simulink model "AKZkz"  (Simulink 4.00)
settings: Solver=ode23tb  StartTime=0.0  StopTime=1
InitFcn:
  | powericon('psbinitsys',bdroot);
libraries: powerlib2 x3, powerlib_extras x3
settings Model: LastModifiedBy=ieao  BlockReductionOpt=off

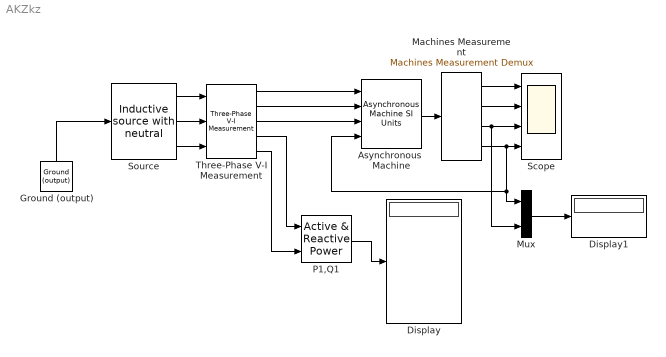
== system AKZkz ==
  "Asynchronous  Machine " : powerlib2/Machines/Asynchronous Machine SI Units  Tag=PoWeRsYsTeMbLoCk  rotType=Squirrel-cage  ctrl=Stationary  x1=[2e3, 380 50 ]  x2="[ 0.435  2.0e-3 ]"  x3="[ 0.816  2.0e-3 ]"  x4=69.31e-3  x5="[ 0.089  0  2 ]"  x6="[ 1,0   0,0,0   0,0,0 ]"  PSBOutputType=1110  iounits=1
  Display : Display
      settings: Format=short
  Display1 : Display
      settings: Format=short
  Ground (output) : powerlib2/Connectors/Ground (output)  Tag=PoWeRsYsTeMbLoCk  Orientation=up  PSBOutputType=1
  Machines Measurement : powerlib2/Machines/Machines Measurement Demux  machType=Asynchronous  ssm1=on  ssm2=on  ssm3=on  ssm4=on  ssm5=on  ssm6=on  sm1=on  sm2=on  sm3=on  sm4=on  sm5=on  sm6=on  sm7=on  sm8=on  sm9=on  sm10=on  sm11=on  asm1=on  asm2=off  asm3=off  asm4=off  asm5=on  asm6=off  asm7=off  asm8=off  asm9=on  asm10=on  asm11=off  pmsm1=on  pmsm2=on  pmsm3=on  pmsm4=on  pmsm5=on  pmsm6=on  lastType=1
  Mux : Mux  Inputs=2
      settings: DisplayOption=none
  P1,Q1 : powerlib_extras/Measurements/Active & Reactive Power  f1=50
  Scope : Scope  NumInputPorts=4
      settings: TimeRange=auto  YMin=-5~-5~-5~-5  YMax=5~5~5~5  SaveToWorkspace=off  SaveName=ScopeData  MaxDataPoints=5000
  Source : powerlib_extras/Three-Phase Library/Inductive source with neutral  V=310  Phi=0  F=50  R=0.724  L=0
  Three-Phase V-I Measurement : powerlib_extras/Measurements/Three-Phase V-I Measurement  phaseurs=off  Vpu=off  Vbase=500e3  Ppu=off  Pbase=100e6
  wires:
  "Asynchronous  Machine "/1 -> Machines Measurement/1
  Source/1 -> Three-Phase V-I Measurement/1
  Source/2 -> Three-Phase V-I Measurement/2
  Source/3 -> Three-Phase V-I Measurement/3
  Three-Phase V-I Measurement/1 -> "Asynchronous  Machine "/1
  Three-Phase V-I Measurement/2 -> "Asynchronous  Machine "/2
  Three-Phase V-I Measurement/3 -> "Asynchronous  Machine "/3
  Three-Phase V-I Measurement/4 -> P1,Q1/1
  Three-Phase V-I Measurement/5 -> P1,Q1/2
  P1,Q1/1 -> Display/1
  Machines Measurement/1 -> Scope/1
  Ground (output)/1 -> Source/1
  Machines Measurement/2 -> Scope/2
  Machines Measurement/3 -> Scope/3, Mux/2
  Machines Measurement/4 -> Scope/4, Mux/1, "Asynchronous  Machine "/4
  Mux/1 -> Display1/1
